simulink model "Concatenate_TestGen12"  (R2017b)
settings: Solver=FixedStepDiscrete  StartTime=0.0  StopTime=10.0  RelTol=1e-3
undefined symbols (not defined in the file): Block_TestLib, trigger
settings Model: Creator=ktrinh  LastModifiedBy=ktrinh
settings DebuggingCC: ParameterOverflowMsg=none

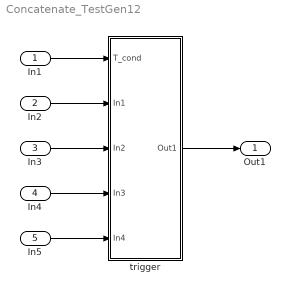
== system Concatenate_TestGen12 ==
  In1 : Inport
  In2 : Inport  Port=2
  In3 : Inport  Port=3
  In4 : Inport  Port=4
  In5 : Inport  Port=5
  trigger : Subsystem  AncestorBlock=Block_TestLib/trigger
  Out1 : Outport
  wires:
  In1/1 -> trigger/1(T_cond)
  In2/1 -> trigger/2(In1)
  In3/1 -> trigger/3(In2)
  In4/1 -> trigger/4(In3)
  In5/1 -> trigger/5(In4)
  trigger/1(Out1) -> Out1/1

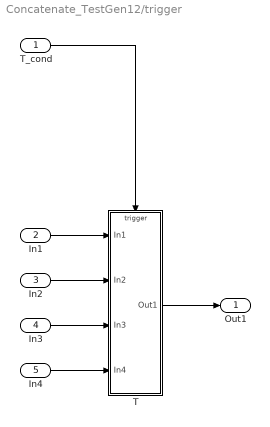
== system Concatenate_TestGen12/trigger ==
  T_cond : Inport  OutDataTypeStr=boolean
  In1 : Inport  Port=2
  In2 : Inport  Port=3
  In3 : Inport  Port=4
  In4 : Inport  Port=5
  T : Subsystem  TreatAsAtomicUnit=on
  Out1 : Outport
  wires:
  T_cond/1 -> T/Trigger
  In1/1 -> T/1(In1)
  In2/1 -> T/2(In2)
  In3/1 -> T/3(In3)
  In4/1 -> T/4(In4)
  T/1(Out1) -> Out1/1

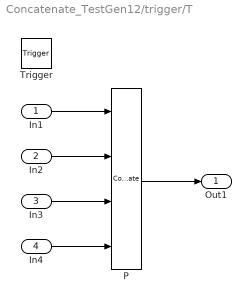
== system Concatenate_TestGen12/trigger/T ==
  In1 : Inport  OutDataTypeStr=int16  PortDimensions=[2 4 5]
  In2 : Inport  Port=2  OutDataTypeStr=int16  PortDimensions=[2 4 5]
  In3 : Inport  Port=3  OutDataTypeStr=int16  PortDimensions=[2 4 5]
  In4 : Inport  Port=4  OutDataTypeStr=int16  PortDimensions=[2 4 5]
  Trigger : TriggerPort  VariantControl=Variant
  P : Concatenate  NumInputs=4  Mode=Multidimensional array  ConcatenateDimension=2
  Out1 : Outport
  wires:
  In1/1 -> P/1
  In2/1 -> P/2
  In3/1 -> P/3
  In4/1 -> P/4
  P/1 -> Out1/1
